simulink model "System_20220515"  (R2020b)
settings: Solver=ode4  StartTime=0.0  StopTime=inf  FixedStep=Ts  RelTol=1e-3  EnableMultiTasking=on
PreLoadFcn:
  | simulation_vars
PostLoadFcn:
  | simulation_vars
InitFcn:
  | simulation_vars
StartFcn:
  | simulation_vars
values from neighbouring files (symbols this model uses):
  ang_variance = 0.001*60    (= 0.06)    [simulation_vars.m]
  bus_va_seed = abs(round(1000*randn(73,1)))    [simulation_vars.m]
  bus_vm_seed = abs(round(1000*randn(73,1)))    [simulation_vars.m]
  event_time_end = event_time_start + 5/60    (= 10000.0833333)    [simulation_vars.m]
  event_time_start = 10000    [simulation_vars.m]
  line_iang0_seed = abs(round(1000*randn(104,1)))    [simulation_vars.m]
  line_iang1_seed = abs(round(1000*randn(104,1)))    [simulation_vars.m]
  line_imag0_seed = abs(round(1000*randn(104,1)))    [simulation_vars.m]
  line_imag1_seed = abs(round(1000*randn(104,1)))    [simulation_vars.m]
  mag_variance = 0.0005    [simulation_vars.m]
  spoof_lower_limit = -pi()/9    [simulation_vars.m]
  spoof_upper_limit = pi()/9    [simulation_vars.m]
  Ts = 0.001    [simulation_vars.m]
  xf_iang0_seed = abs(round(1000*randn(16,1)))    [simulation_vars.m]
  xf_iang1_seed = abs(round(1000*randn(16,1)))    [simulation_vars.m]
  xf_imag0_seed = abs(round(1000*randn(16,1)))    [simulation_vars.m]
  xf_imag1_seed = abs(round(1000*randn(16,1)))    [simulation_vars.m]
undefined symbols (not defined in the file or in its folder): en_spoofing_attack
libraries: rtlab x210, simulink x21, opal_lib x1, rtlab_phasor x1, rtio_spectracom x1
(part 1 of 4)
Description:
  | Model of a simple control system for use iin training.
settings Model: Creator=Paul Baracos  LastModifiedBy=sudo
settings DataIOCC: LimitDataPoints=on  SaveFormat=Array  SignalLoggingSaveFormat=ModelDataLogs  SaveOutput=off  SaveTime=off  ReturnWorkspaceOutputs=off  SignalLoggingName=sigsOut
settings OptimizationCC: BlockReduction=off  BooleanDataType=off  OptimizeBlockIOStorage=off  BufferReuse=off  ExpressionFolding=off  LocalBlockOutputs=off  InitFltsAndDblsToZero=on  LifeSpan=inf
settings DebuggingCC: SaveWithParameterizedLinksMsg=none  UnderspecifiedInitializationDetection=Classic  MergeDetectMultiDrivingBlocksExec=none  SignalResolutionControl=TryResolveAllWithWarning  MultiTaskDSMMsg=warning  MultiTaskCondExecSysMsg=none  FcnCallInpInsideContextMsg=warning  SFUnexpectedBacktrackingDiag=warning  SFNoUnconditionalDefaultTransitionDiag=warning  SFExecutionAtInitializationDiag=none  ArithmeticOperatorsInVariantConditions=warning
settings HardwareCC: ProdBitPerPointer=32  ProdBitPerSizeT=32  ProdBitPerPtrDiffT=32  ProdLargestAtomicFloat=None  ProdIntDivRoundTo=Undefined  ProdEndianess=Unspecified  ProdWordSize=32  ProdHWDeviceType=32-bit Generic  TargetUnknown=on
settings ModelReferenceCC: PropagateSignalLabelsOutOfModel=off
settings SFSimCC: SimUseLocalCustomCode=off  CustomCodeUndefinedFunction=UseInterfaceOnly
settings RTWCC: RTWUseLocalCustomCode=off
settings CodeAppCC: StateflowObjectComments=on
settings GRTTargetCC: TargetFcnLib=ansi_tfl_tmw.mat  TargetLangStandard=C89/C90 (ANSI)  CombineOutputUpdateFcns=off  GRTInterface=on
settings ConfigComp: CovMetricSettings=dw  CovSaveCumulativeToWorkspaceVar=on  CovSaveSingleToWorkspaceVar=on  CovExternalEMLEnable=off

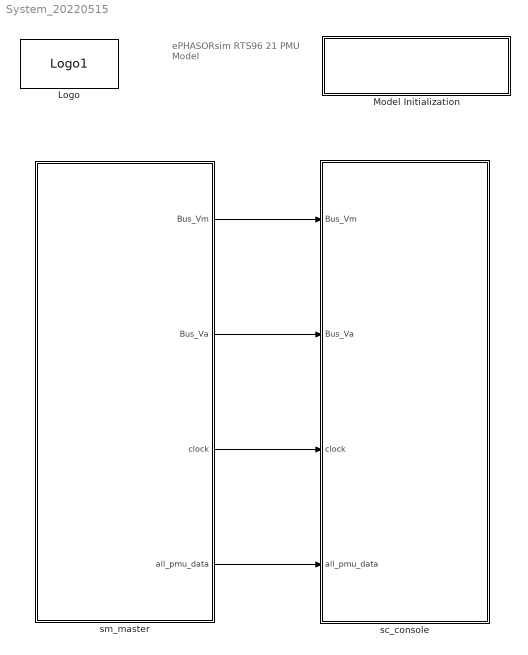
== system System_20220515 ==
  note: ePHASORsim
      | RTS96
      | 21 PMU Model
  Logo : opal_lib/Logo1  vide=[]
  Model Initialization : Subsystem  mask(Model Functions){InitFcnX=simulation_vars, prel=on, posl=on, inif=on, strf=on}
      mask prompts: InitFcnX "Initialisation"; prel "Preload Function"; posl "PostLoad Function"; inif "InitFcn"; strf "StartFcn"
      mask init:
      | currentBlock = gcb;
      | root = bdroot(currentBlock);
      | 
      | if ~strcmp(get_param(root,'BlockDiagramType'),'library')
      |     if prel==1
      |         set_param(root, 'PreLoadFcn', InitFcnX);
      |     else
      |         set_param(root, 'PreLoadFcn', '');
      |     end
      |     if inif==1
      |         set_param(root, 'InitFcn', InitFcnX);
      |     else
      |         set_param(root, 'InitFcn', '');
      |     end
      |     if strf==1
      |         set_param(root, 'StartFcn', InitFcnX);
      |     else
      |         set_param(root, 'StartFcn', '');
      |     end
      |     if posl==1
      |         set_param(root, 'PostLoadFcn', InitFcnX);
      |     else
      |         set_param(root, 'PostLoadFcn', '');
      |     end
      | end
      | 
      | pos = get_param(currentBlock, 'Position');
      | width = pos(3) - pos(1); height = pos(4) - pos(2);
      | txt = [ upper(root) '\n' '- InitFcn. . . . . '  get_param(root, 'InitFcn') ];
      settings: CopyFcn=set_param(gcb,'LinkStatus','none')
      mask Display: text(5, height*0.5, txt, 'horizontalAlignment', 'left', 'verticalAlignment', 'middle') ;
  sc_console : Subsystem
  sm_master : Subsystem
  wires:
  sm_master/1(Bus_Vm) -> sc_console/1(Bus_Vm)
  sm_master/3(clock) -> sc_console/3(clock)
  sm_master/4(all_pmu_data) -> sc_console/4(all_pmu_data)
  sm_master/2(Bus_Va) -> sc_console/2(Bus_Va)

== system System_20220515/Model Initialization ==

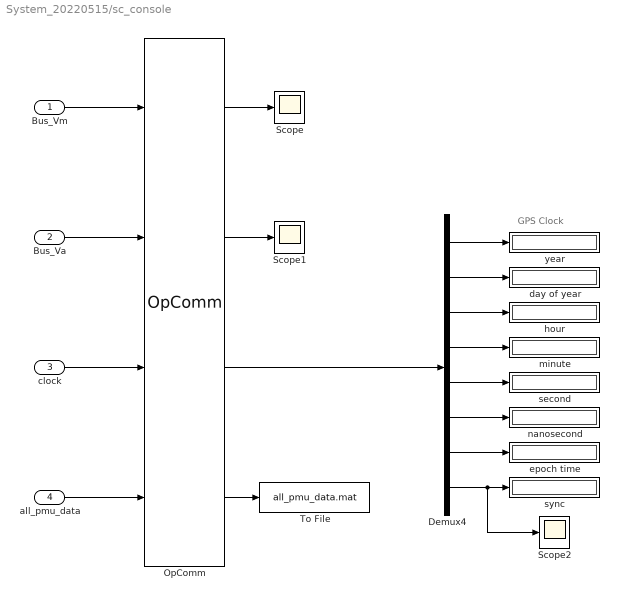
== system System_20220515/sc_console ==
  note: GPS Clock
  Bus_Vm : Inport
  Bus_Va : Inport  Port=2
  clock : Inport  Port=3
  all_pmu_data : Inport  Port=4
  Demux4 : Demux  Outputs=8
  OpComm : rtlab/OpComm  nbport=4  groupe_acq=1  subsys_rate=0  st=0  Synchronization=on  Interpolation=on  Threshold=1.0  Missed_Data=off  Sim_Time=off  Samples=off  dynSigOut=off  from_console=0  warning_done=off  writeOpCommFile=off  Offset=off
      settings: SourceProductName=RT-LAB
  Scope : Scope
  Scope1 : Scope
  Scope2 : Scope
  To File : ToFile  Filename=all_pmu_data.mat  SaveFormat=Timeseries
  day of year : Display
  epoch time : Display
  hour : Display
  minute : Display
  nanosecond : Display
  second : Display
  sync : Display
  year : Display
  wires:
  Bus_Vm/1 -> OpComm/1
  OpComm/1 -> Scope/1
  Demux4/3 -> hour/1
  Demux4/8 -> Scope2/1, sync/1
  Demux4/4 -> minute/1
  Demux4/2 -> day of year/1
  Demux4/5 -> second/1
  Demux4/6 -> nanosecond/1
  Demux4/1 -> year/1
  Demux4/7 -> epoch time/1
  all_pmu_data/1 -> OpComm/4
  clock/1 -> OpComm/3
  Bus_Va/1 -> OpComm/2
  OpComm/4 -> To File/1
  OpComm/3 -> Demux4/1
  OpComm/2 -> Scope1/1

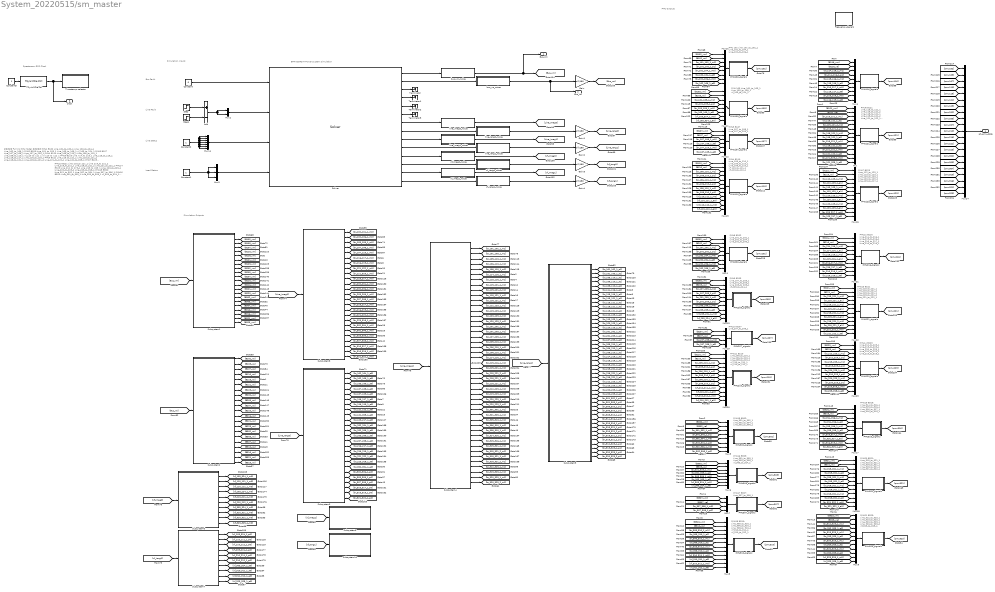
== system System_20220515/sm_master ==
  note: PMU13 B221
      | Line_215_to_221_1
      | Line_215_to_221_2
      | Line_218_to_221_1
      | Line_218_to_221_2
      | Line_221_to_222_1
      |
      | PMU14 B223
      | Line_212_to_223_1
      | Line_213_to_223_1
      | Line_220_to_223_1
      | Line_220_to_223_2
      | Line_223_to_318_1
      |
      | PMU15 B302:
      | Line_301_to_302_1
      | Line_302_to_304_1
      | Line_302_to_306_1
      |
      | PMU16 B303:
      | Line_301_to_303_1
      | Line_303_to_309_1
      | xf_303_to_324_1
      |
      | PMU17 B307:
      | Line_307_to_308_1
      |
      | PMU18 B310:
      | Line_305_to_310_1
      | Line_306_to_310_1
      | Line_308_to_310_1
      | xf_310_to_311_1
      | xf_310_to_312_1
      |
      | PMU19 B316:
      | Line_314_to_316_1
      | Line_315_to_316_1
      | Line_316_to_317_1
      | Line_316_to_319_1
      |
      | PMU20 B321:
      | Line_315_to_321_1
      | Line_315_to_321_2
      | Line_318_to_321_1
      | Line_318_to_321_2
      | Line_321_to_322_1
      |
      | PMU21 B323:
      | Line_312_to_323_1
      | Line_313_to_323_1
      | Line_320_to_323_1
      | Line_320_to_323_2
      | xf_323_to_325_1
  note: PMU14 B223
      | Line_212_to_223_1
      | Line_213_to_223_1
      | Line_220_to_223_1
      | Line_220_to_223_2
      | Line_223_to_318_1
  note: PMU12 B216
      | Line_214_to_216_1
      | Line_215_to_216_1
      | Line_216_to_217_1
      | Line_216_to_219_1
  note: PMU11 B210
      | Line_205_to_210_1
      | Line_206_to_210_1
      | Line_208_to_210_1
      | xf_210_to_211_1
      | xf_210_to_212_1
  note: PMU10 B207
      | Line_207_to_208_1
  note: PMU9 B203
      | Line_107_to_203_1
      | Line_201_to_203_1
      | Line_203_to_209_1
      | xf_203_to_224_1
  note: PMU8 B202
      | Line_201_to_202_1
      | LIne_202_to_204_1
      | Line_202_to_206_1
  note: PMU21 B323:
      | Line_312_to_323_1
      | Line_313_to_323_1
      | Line_320_to_323_1
      | Line_320_to_323_2
      | xf_323_to_325_1
  note: PMU20 B321:
      | Line_315_to_321_1
      | Line_315_to_321_2
      | Line_318_to_321_1
      | Line_318_to_321_2
      | Line_321_to_322_1
  note: PMU19 B316:
      | Line_314_to_316_1
      | Line_315_to_316_1
      | Line_316_to_317_1
      | Line_316_to_319_1
  note: PMU18 B310:
      | Line_305_to_310_1
      | Line_306_to_310_1
      | Line_308_to_310_1
      | xf_310_to_311_1
      | xf_310_to_312_1
  note: PMU17 B307:
      | Line_307_to_308_1
  note: PMU16 B303:
      | Line_301_to_303_1
      | Line_303_to_309_1
      | xf_303_to_324_1
  note: PMU15 B302:
      | Line_301_to_302_1
      | Line_302_to_304_1
      | Line_302_to_306_1
  note: PMU 102
      | Line_101_to_102_1
      | Line_102_to_104_1
      | Line_102_to_106_1
  note: EPHASORSIM Power System Simulation
  note: Simulation Inputs
  note: Simulation Outputs
  note: PMU Outputs
  note: Spectracom GPS Clock
  note: ##### Full 21 PMU Model #####
      | PMU1 B102
      | Line_101_to_102_1
      | Line_102_to_104_1
      | Line_102_to_106_1
      |
      | PMU2 B103
      | Line_101_to_103_1
      | Line_103_to_109_1
      | xf_103_to_124_1
      |
      | PMU3 B107
      | Line_107_to_108_1
      | Line_107_to_203_1
      |
      | PMU4 B110
      | Line_105_to_110_1
      | Line_106_to_110_1
      | Line_108_to_110_1
      | xf_110_to_111_1
      | xf_110_to_112_1
      |
      | PMU5 B116
      | Line_114_to_116_1
      | Line_115_to_116_1
      | Line_116_to_117_1
      | Line_116_to_119_1
      |
      | PMU6 B121
      | Line_115_to_121_1
      | Line_115_to_121_2
      | Line_118_to_121_1
      | Line_118_to_121_2
      | Line_121_to_122_1
      | Line_121_to_325_1
      |
      | PMU7 B123
      | Line_112_to_123_1
      | Line_113_to_123_1
      | Line_120_to_123_1
      | Line_120_to_123_2
      | Line_123_to_217_1
      |
      | PMU8 B202
      | Line_201_to_202_1
      | LIne_202_to_204_1
      | Line_202_to_206_1
      |
      | PMU9 B203
      | Line_201_to_203_1
      | Line_203_to_209_1
      | Line_107_to_203_1
      | xf_203_to_224_1
      |
      | PMU10 B207
      | Line_207_to_208_1
      |
      | PMU11 B210
      | Line_205_to_210_1
      | Line_206_to_210_1
      | Line_208_to_210_1
      | xf_210_to_211_1
      | xf_210_to_212_1
      |
      | PMU12 B216
      | Line_214_to_216_1
      | Line_215_to_216_1
      | Line_216_to_217_1
      | Line_216_to_219_1
  note: Bus Fault
  note: Line Fault
  note: Line Status
  note: Load Status
  note: PMU 103
      | Line_101_to_103_1
      | Line_103_to_109_1
      | xf_103_to_124_1
  note: PMU3 B107
      | Line_107_to_108_1
      | Line_107_to_203_1
  note: PMU4 B110
      | Line_105_to_110_1
      | Line_106_to_110_1
      | Line_108_to_110_1
      | xf_110_to_111_1
      | xf_110_to_112_1
  note: PMU6 B121
      | Line_115_to_121_1
      | Line_115_to_121_2
      | Line_118_to_121_1
      | Line_118_to_121_2
      | Line_121_to_122_1
      | Line_121_to_325_1
  note: PMU7 B123
      | Line_112_to_123_1
      | Line_113_to_123_1
      | Line_120_to_123_1
      | Line_120_to_123_2
      | Line_123_to_217_1
  note: PMU13 B221
      | Line_215_to_221_1
      | Line_215_to_221_2
      | Line_218_to_221_1
      | Line_218_to_221_2
      | Line_221_to_222_1
  Add : Sum  Inputs=+-
  Constant : Constant  Value=0
  Constant1 : Constant
  Constant2 : Constant
  Constant3 : Constant
  Frequency_signals : Subsystem
  Gain{,1..4} (5 alike) : Gain  Gain=pi()/180
  Mux : Mux  Inputs=14
  Mux{1,5..6,10..11} (5 alike) : Mux  Inputs=8
  Mux12 : Mux  Inputs=6
  Mux{4,13,17,21} (4 alike) : Mux  Inputs=10
  Mux14 : Mux  Inputs=7
  Mux{8..9,15..16,18,20,22..23} (8 alike) : Mux  Inputs=12
  Mux19 : Mux
  Mux2 : Mux  Inputs=2
  Mux24 : Mux  Inputs=21
  Mux3 : Mux  Inputs=3
  Mux7 : Mux
  PMU102_signals : Subsystem
  PMU103_signals : Subsystem
  PMU107_signals : Subsystem
  PMU110_signals : Subsystem
  PMU116_signals : Subsystem
  PMU121_signals : Subsystem
  PMU123_signals : Subsystem
  PMU202_signals : Subsystem
  PMU203_signals : Subsystem
  PMU207_signals : Subsystem
  PMU210_signals : Subsystem
  PMU216_signals : Subsystem
  PMU221_signals : Subsystem
  PMU223_signals : Subsystem
  PMU302_signals : Subsystem
  PMU303_signals : Subsystem
  PMU307_signals : Subsystem
  PMU310_signals : Subsystem
  PMU316_signals : Subsystem
  PMU321_signals : Subsystem
  PMU323_signals : Subsystem
  Solver : rtlab_phasor/Solver  epname=System  extension=PSS/e Ver. 32  use_udb=off  xls='RTS96_pins_simple_v2.xls'  raw='RTS96_psse_stable.raw'  dyr='Dynamics.dyr'  fmu2builtin=off  cyme='typical.sxst'  cyme_pf=''  cyme_unbalanced=on  powerfactory='network.dgs'  builtin=on  lazy_netlist=on  capidir='CAPI'  fmudir='FMU'  capiprefix=capicomp_  fmuprefix=fmucomp_  logging=off  sim_mode=Power-flow and dynamic simulation  dt=Ts  pf_init_method=From input data  pf_tol_v=0.00000001  pf_max_it=100  pf_smart_start=off  pf_flat_start=off  pf_export=off  pfrequest=off  pf_then_dyn=on  np=1  exporty=off  optim_threads=on  perflog_on=off  script_activate_postinit=off  script_postinit_name=''
  Step : Step  Time=event_time_start  SampleTime=0
  Step1 : Step  Time=event_time_end  SampleTime=0
  Subsystem1 : Subsystem
  Subsystem10 : Subsystem
  Subsystem2 : Subsystem
  Subsystem3 : Subsystem
  Subsystem4 : Subsystem
  Subsystem5 : Subsystem
  Subsystem6 : Subsystem
  Subsystem7 : Subsystem
  Subsystem8 : Subsystem
  Subsystem9 : Subsystem
  TSync PCIe Ctrl : rtio_spectracom/TSync PCIe Ctrl  devIx=0  holdover_timeout=5  timestamp_en=on  set_time_en=off  ts_wo_sync_opt=UTC 0
  Terminator{,1..3} (4 alike) : Terminator
  Timestamp selector : Subsystem
  bus_va_noise : Subsystem
  bus_vm_noise : Subsystem
  line_iang0_noise : Subsystem
  line_iang1_noise : Subsystem
  line_imag0_noise : Subsystem
  line_imag1_noise : Subsystem
  xf_iang0_noise : Subsystem
  xf_iang1_noise : Subsystem
  xf_imag0_noise : Subsystem
  xf_imag1_noise : Subsystem
  Bus_Vm : Outport  VectorParamsAs1DForOutWhenUnconnected=off
  Bus_Va : Outport  Port=2
  clock : Outport  Port=3
  all_pmu_data : Outport  Port=4
  wires:
  Solver/2 -> bus_va_noise/1(In1)
  Solver/10 -> line_iang1_noise/1(In1)
  Solver/8 -> line_iang0_noise/1(In1)
  Solver/12 -> xf_iang0_noise/1(In1)
  Subsystem1/5(B116_Vmag) -> [B116_vm]
  Subsystem1/16(B303_Vmag) -> [B303_vm]
  Subsystem1/6(B121_Vmag) -> [B121_vm]
  Subsystem1/17(B307_Vmag) -> [B307_vm]
  Subsystem1/15(B302_Vmag) -> [B302_vm]
  Subsystem1/18(B310_Vmag) -> [B310_vm]
  Subsystem1/21(B323_Vmag) -> [B323_vm]
  Subsystem2/15(B302_Vang) -> [B302_va]
  Subsystem2/6(B121_Vang) -> [B121_va]
  Subsystem2/5(B116_Vang) -> [B116_va]
  Subsystem2/16(B303_Vang) -> [B303_va]
  Subsystem2/17(B307_Vang) -> [B307_va]
  Subsystem2/18(B310_Vang) -> [B310_va]
  Subsystem2/21(B323_Vang) -> [B323_va]
  Subsystem4/6(Line_114_to_116_1_mag) -> [br_114_116_1_m1]
  Subsystem4/7(Line_115_to_116_1_mag) -> [br_115_116_1_m1]
  Subsystem8/6(Line_116_to_117_1_mag) -> [br_116_117_1_m0]
  Subsystem8/7(Line_116_to_119_1_mag) -> [br_116_119_1_m0]
  Subsystem4/8(Line_115_to_121_1_mag) -> [br_115_121_1_m1]
  Subsystem4/9(Line_115_to_121_2_mag) -> [br_115_121_2_m1]
  Subsystem4/10(Line_118_to_121_1_mag) -> [br_118_121_1_m1]
  Subsystem4/11(Line_118_to_121_2_mag) -> [br_118_121_2_m1]
  Subsystem8/8(Line_121_to_122_1_mag) -> [br_121_122_1_m0]
  Subsystem8/9(Line_121_to_325_1_mag) -> [br_121_325_1_m0]
  Subsystem4/32(Line_301_to_302_1_mag) -> [br_301_302_1_m1]
  Subsystem8/19(Line_302_to_304_1_mag) -> [br_302_304_1_m0]
  Subsystem8/20(Line_302_to_306_1_mag) -> [br_302_306_1_m0]
  Subsystem4/33(Line_301_to_303_1_mag) -> [br_301_303_1_m1]
  Subsystem8/21(Line_303_to_309_1_mag) -> [br_303_309_1_m0]
  Subsystem8/22(Line_307_to_308_1_mag) -> [br_307_308_1_m0]
  Subsystem4/34(Line_305_to_310_1_mag) -> [br_305_310_1_m1]
  Subsystem4/35(Line_306_to_310_1_mag) -> [br_306_310_1_m1]
  Subsystem4/36(Line_308_to_310_1_mag) -> [br_308_310_1_m1]
  Subsystem4/43(Line_312_to_323_1_mag) -> [br_312_323_1_m1]
  Subsystem4/44(Line_313_to_323_1_mag) -> [br_313_323_1_m1]
  Subsystem4/45(Line_320_to_323_1_mag) -> [br_320_323_1_m1]
  Subsystem4/46(Line_320_to_323_2_mag) -> [br_320_323_2_m1]
  Subsystem6/7(xf_303_to_324_1_mag) -> [xf_303_324_1_m0]
  Subsystem6/8(xf_310_to_311_1_mag) -> [xf_310_311_1_m0]
  Subsystem6/9(xf_310_to_312_1_mag) -> [xf_310_312_1_m0]
  Subsystem6/10(xf_323_to_325_1_mag) -> [xf_323_325_1_m0]
  Solver/14 -> xf_iang1_noise/1(In1)
  Constant/1 -> Solver/1
  Step/1 -> Add/1
  Step1/1 -> Add/2
  Mux2/1 -> Solver/2
  Add/1 -> Mux2/1, Mux2/2
  Mux3/1 -> Solver/4
  Constant1/1 -> Mux3/3, Mux3/1, Mux3/2
  Mux14/1 -> Solver/3
  [B116_vm] -> Mux4/1
  [B116_va] -> Mux4/2
  [br_114_116_1_m1] -> Mux4/3
  [br_114_116_1_a1] -> Mux4/4
  [br_115_116_1_m1] -> Mux4/5
  [br_115_116_1_a1] -> Mux4/6
  [br_116_117_1_m0] -> Mux4/7
  [br_116_117_1_a0] -> Mux4/8
  [br_116_119_1_m0] -> Mux4/9
  [br_116_119_1_a0] -> Mux4/10
  [B121_vm] -> Mux/1
  [B121_va] -> Mux/2
  [br_115_121_1_m1] -> Mux/3
  Mux/1 -> PMU121_signals/1(In1)
  [br_115_121_1_a1] -> Mux/4
  [br_115_121_2_m1] -> Mux/5
  [br_115_121_2_a1] -> Mux/6
  [br_118_121_1_m1] -> Mux/7
  [br_118_121_1_a1] -> Mux/8
  [br_118_121_2_m1] -> Mux/9
  [br_118_121_2_a1] -> Mux/10
  [br_121_122_1_m0] -> Mux/11
  [br_121_122_1_a0] -> Mux/12
  [br_121_325_1_m0] -> Mux/13
  [br_121_325_1_a0] -> Mux/14
  Mux5/1 -> PMU302_signals/1(In1)
  [B302_vm] -> Mux5/1
  [B302_va] -> Mux5/2
  [br_301_302_1_m1] -> Mux5/3
  [br_301_302_1_a1] -> Mux5/4
  [br_302_304_1_m0] -> Mux5/5
  [br_302_304_1_a0] -> Mux5/6
  [br_302_306_1_m0] -> Mux5/7
  [br_302_306_1_a0] -> Mux5/8
  [B303_vm] -> Mux6/1
  [B303_va] -> Mux6/2
  [br_301_303_1_m1] -> Mux6/3
  [br_301_303_1_a1] -> Mux6/4
  [br_303_309_1_m0] -> Mux6/5
  [br_303_309_1_a0] -> Mux6/6
  [xf_303_324_1_m0] -> Mux6/7
  [xf_303_324_1_a0] -> Mux6/8
  Mux6/1 -> PMU303_signals/1(In1)
  [B307_vm] -> Mux7/1
  [B307_va] -> Mux7/2
  [br_307_308_1_m0] -> Mux7/3
  [br_307_308_1_a0] -> Mux7/4
  Mux7/1 -> PMU307_signals/1(In1)
  [B310_vm] -> Mux8/1
  [B310_va] -> Mux8/2
  [br_305_310_1_m1] -> Mux8/3
  [br_305_310_1_a1] -> Mux8/4
  [br_306_310_1_m1] -> Mux8/5
  [br_306_310_1_a1] -> Mux8/6
  [br_308_310_1_m1] -> Mux8/7
  [br_308_310_1_a1] -> Mux8/8
  [xf_310_311_1_m0] -> Mux8/9
  [xf_310_311_1_a0] -> Mux8/10
  [xf_310_312_1_m0] -> Mux8/11
  [xf_311_312_1_a0] -> Mux8/12
  Mux8/1 -> PMU310_signals/1(In1)
  [B323_vm] -> Mux9/1
  [B323_va] -> Mux9/2
  [br_312_323_1_m1] -> Mux9/3
  [br_312_323_1_a1] -> Mux9/4
  [br_313_323_1_m1] -> Mux9/5
  [br_313_323_1_a1] -> Mux9/6
  [br_320_323_1_m1] -> Mux9/7
  [br_320_323_1_a1] -> Mux9/8
  [br_320_323_2_m1] -> Mux9/9
  [br_320_323_2_a1] -> Mux9/10
  [xf_323_325_1_m0] -> Mux9/11
  [xf_323_325_1_a0] -> Mux9/12
  Mux9/1 -> PMU323_signals/1(In1)
  PMU121_signals/1(Out1) -> [pmu121]
  PMU302_signals/1(Out1) -> [pmu302]
  PMU303_signals/1(Out1) -> [pmu303]
  PMU307_signals/1(Out1) -> [pmu307]
  PMU310_signals/1(Out1) -> [pmu310]
  PMU323_signals/1(Out1) -> [pmu323]
  PMU116_signals/1(Out1) -> [pmu116]
  Mux4/1 -> PMU116_signals/1(In1)
  TSync PCIe Ctrl/1 -> clock/1, Timestamp selector/1(ts_in)
  Constant3/1 -> TSync PCIe Ctrl/1
  Constant2/1 -> Mux14/5, Mux14/7, Mux14/6, Mux14/1, Mux14/2, Mux14/3, Mux14/4
  Solver/3 -> Terminator/1
  Solver/4 -> Terminator1/1
  Solver/5 -> Terminator2/1
  Solver/6 -> Terminator3/1
  Subsystem1/1(B102_Vmag) -> [B102_vm]
  [B102_vm] -> Mux10/1
  Subsystem2/1(B102_Vang) -> [B102_va]
  [B102_va] -> Mux10/2
  Mux10/1 -> PMU102_signals/1(In1)
  PMU102_signals/1(Out1) -> [pmu102]
  Subsystem4/1(Line_101_to_102_1_mag) -> [br_101_102_1_m1]
  [br_101_102_1_m1] -> Mux10/3
  [br_101_102_1_a1] -> Mux10/4
  Subsystem8/2(Line_102_to_106_1_mag) -> [br_102_106_1_m0]
  Subsystem8/1(Line_102_to_104_1_mag) -> [br_102_104_1_m0]
  [br_102_104_1_m0] -> Mux10/5
  [br_102_106_1_m0] -> Mux10/7
  Gain1/1 -> [Line_Iang0]
  [Line_Imag0] -> Subsystem8/1(Imag0)
  [Line_Iang0] -> Subsystem3/1(Iang0)
  Gain2/1 -> [Line_Iang1]
  [Line_Imag1] -> Subsystem4/1(Imag1)
  [Line_Iang1] -> Subsystem5/1(Iang1)
  [xf_Imag0] -> Subsystem6/1(Imag0)
  Gain3/1 -> [xf_Iang0]
  [xf_Iang0] -> Subsystem7/1(Iang0)
  [xf_Imag1] -> Subsystem9/1(Imag1)
  Gain4/1 -> [xf_Iang1]
  [Bus_vm] -> Subsystem1/1(bus_vm)
  Gain/1 -> [Bus_va]
  [Bus_va] -> Subsystem2/1(bus_va)
  Subsystem3/6(Line_116_to_117_1_ang) -> [br_116_117_1_a0]
  Subsystem3/7(Line_116_to_119_1_ang) -> [br_116_119_1_a0]
  Subsystem3/8(Line_121_to_122_1_ang) -> [br_121_122_1_a0]
  Subsystem3/9(Line_121_to_325_1_ang) -> [br_121_325_1_a0]
  Subsystem3/22(Line_307_to_308_1_ang) -> [br_307_308_1_a0]
  Subsystem3/21(Line_303_to_309_1_ang) -> [br_303_309_1_a0]
  Subsystem3/20(Line_302_to_306_1_ang) -> [br_302_306_1_a0]
  Subsystem3/19(Line_302_to_304_1_ang) -> [br_302_304_1_a0]
  Subsystem3/2(Line_102_to_106_1_ang) -> [br_102_106_1_a0]
  Subsystem3/1(Line_102_to_104_1_ang) -> [br_102_104_1_a0]
  [br_102_104_1_a0] -> Mux10/6
  [br_102_106_1_a0] -> Mux10/8
  Subsystem1/2(B103_Vmag) -> [B103_vm]
  Subsystem2/2(B103_Vang) -> [B103_va]
  Subsystem8/3(Line_103_to_109_1_mag) -> [br_103_109_1_m0]
  Subsystem3/3(Line_103_to_109_1_ang) -> [br_103_109_1_a0]
  [xf_Iang1] -> Subsystem10/1(Iang1)
  Subsystem7/7(xf_303_to_324_1_ang) -> [xf_303_324_1_a0]
  Subsystem7/8(xf_310_to_311_1_ang) -> [xf_310_311_1_a0]
  Subsystem7/9(xf_310_to_312_1_ang) -> [xf_311_312_1_a0]
  Subsystem7/10(xf_323_to_325_1_ang) -> [xf_323_325_1_a0]
  Subsystem4/2(Line_101_to_103_1_mag) -> [br_101_103_1_m1]
  Subsystem5/1(Line_101_to_102_1_ang) -> [br_101_102_1_a1]
  Subsystem5/6(Line_114_to_116_1_ang) -> [br_114_116_1_a1]
  Subsystem5/7(Line_115_to_116_1_ang) -> [br_115_116_1_a1]
  Subsystem5/9(Line_115_to_121_2_ang) -> [br_115_121_2_a1]
  Subsystem5/8(Line_115_to_121_1_ang) -> [br_115_121_1_a1]
  Subsystem5/10(Line_118_to_121_1_ang) -> [br_118_121_1_a1]
  Subsystem5/11(Line_118_to_121_2_ang) -> [br_118_121_2_a1]
  Subsystem5/32(Line_301_to_302_1_ang) -> [br_301_302_1_a1]
  Subsystem5/33(Line_301_to_303_1_ang) -> [br_301_303_1_a1]
  Subsystem5/34(Line_305_to_310_1_ang) -> [br_305_310_1_a1]
  Subsystem5/35(Line_306_to_310_1_ang) -> [br_306_310_1_a1]
  Subsystem5/36(Line_308_to_310_1_ang) -> [br_308_310_1_a1]
  Subsystem5/46(Line_320_to_323_2_ang) -> [br_320_323_2_a1]
  Subsystem5/45(Line_320_to_323_1_ang) -> [br_320_323_1_a1]
  Subsystem5/44(Line_313_to_323_1_ang) -> [br_313_323_1_a1]
  Subsystem5/43(Line_312_to_323_1_ang) -> [br_312_323_1_a1]
  Subsystem5/2(Line_101_to_103_1_ang) -> [br_101_103_1_a1]
  [br_101_103_1_m1] -> Mux11/3
  [br_101_103_1_a1] -> Mux11/4
  [br_103_109_1_m0] -> Mux11/5
  [br_103_109_1_a0] -> Mux11/6
  [B103_va] -> Mux11/2
  [B103_vm] -> Mux11/1
  Mux11/1 -> PMU103_signals/1(In1)
  PMU103_signals/1(Out1) -> [pmu103]
  Subsystem1/3(B107_Vmag) -> [B107_vm]
  Subsystem2/3(B107_Vang) -> [B107_va]
  Subsystem8/4(Line_107_to_108_1_mag) -> [br_107_108_1_m0]
  Subsystem3/4(Line_107_to_108_1_ang) -> [br_107_108_1_a0]
  Subsystem8/5(Line_107_to_203_1_mag) -> [br_107_123_1_m0]
  Subsystem3/5(Line_107_to_203_1_ang) -> [br_107_123_1_a0]
  [br_107_123_1_a0] -> Mux12/6
  [br_107_123_1_m0] -> Mux12/5
  [br_107_108_1_a0] -> Mux12/4
  [br_107_108_1_m0] -> Mux12/3
  [B107_va] -> Mux12/2
  [B107_vm] -> Mux12/1
  Mux12/1 -> PMU107_signals/1(In1)
  PMU107_signals/1(Out1) -> [pmu107]
  Subsystem6/1(xf_103_to_124_1_mag) -> [xf_103_324_1_m0]
  [xf_103_324_1_m0] -> Mux11/7
  Subsystem7/1(xf_103_to_124_1_ang) -> [xf_103_324_1_a0]
  [xf_103_324_1_a0] -> Mux11/8
  Subsystem1/4(B110_Vmag) -> [B110_vm]
  Subsystem2/4(B110_Vang) -> [B110_va]
  Subsystem4/3(Line_105_to_110_1_mag) -> [br_105_110_1_m1]
  Subsystem4/4(Line_106_to_110_1_mag) -> [br_106_110_1_m1]
  Subsystem4/5(Line_108_to_110_1_mag) -> [br_108_110_1_m1]
  Subsystem6/2(xf_110_to_111_1_mag) -> [xf_110_111_1_m0]
  Subsystem6/3(xf_110_to_112_1_mag) -> [xf_110_112_1_m0]
  Subsystem7/2(xf_110_to_111_1_ang) -> [xf_110_111_1_a0]
  Subsystem7/3(xf_110_to_112_1_ang) -> [xf_110_112_1_a0]
  Subsystem5/3(Line_105_to_110_1_ang) -> [br_105_110_1_a1]
  Subsystem5/4(Line_106_to_110_1_ang) -> [br_106_110_1_a1]
  Subsystem5/5(Line_108_to_110_1_ang) -> [br_108_110_1_a1]
  [br_108_110_1_m1] -> Mux15/7
  [xf_110_112_1_a0] -> Mux15/12
  Mux15/1 -> PMU110_signals/1(Input)
  [B110_va] -> Mux15/2
  [br_106_110_1_a1] -> Mux15/6
  PMU110_signals/1(Output) -> [pmu110]
  [br_105_110_1_m1] -> Mux15/3
  [xf_110_111_1_m0] -> Mux15/9
  [B110_vm] -> Mux15/1
  [br_108_110_1_a1] -> Mux15/8
  [xf_110_112_1_m0] -> Mux15/11
  [br_105_110_1_a1] -> Mux15/4
  [xf_110_111_1_a0] -> Mux15/10
  [br_106_110_1_m1] -> Mux15/5
  Subsystem1/7(B123_Vmag) -> [B123_vm]
  Subsystem2/7(B123_Vang) -> [B123_va]
  [B123_va] -> Mux16/2
  [B123_vm] -> Mux16/1
  PMU123_signals/1(Out1) -> [pmu123]
  Mux16/1 -> PMU123_signals/1(In1)
  Subsystem8/10(Line_123_to_217_1_mag) -> [br_123_217_1_m0]
  [br_123_217_1_m0] -> Mux16/11
  Subsystem3/10(Line_123_to_217_1_ang) -> [br_123_217_1_a0]
  [br_123_217_1_a0] -> Mux16/12
  Subsystem4/12(Line_112_to_123_1_mag) -> [br_112_123_1_m1]
  Subsystem4/13(Line_113_to_123_1_mag) -> [br_113_123_1_m1]
  Subsystem4/14(Line_120_to_123_1_mag) -> [br_120_123_1_m1]
  Subsystem4/15(Line_120_to_123_2_mag) -> [br_120_123_2_m1]
  [br_113_123_1_m1] -> Mux16/5
  [br_112_123_1_m1] -> Mux16/3
  [br_120_123_1_m1] -> Mux16/7
  [br_120_123_2_m1] -> Mux16/9
  Subsystem5/12(Line_112_to_123_1_ang) -> [br_112_123_1_a1]
  Subsystem5/13(Line_113_to_123_1_ang) -> [br_113_123_1_a1]
  Subsystem5/14(Line_120_to_123_1_ang) -> [br_120_123_1_a1]
  Subsystem5/15(Line_120_to_123_2_ang) -> [br_120_123_2_a1]
  [br_120_123_2_a1] -> Mux16/10
  [br_120_123_1_a1] -> Mux16/8
  [br_113_123_1_a1] -> Mux16/6
  [br_112_123_1_a1] -> Mux16/4
  Subsystem1/19(B316_Vmag) -> [B316_vm]
  Subsystem1/20(B321_Vmag) -> [B321_vm]
  Subsystem1/8(B202_Vmag) -> [B202_vm]
  Subsystem1/9(B203_Vmag) -> [B203_vm]
  Subsystem1/10(B207_Vmag) -> [B207_vm]
  Subsystem1/11(B210_Vmag) -> [B210_vm]
  Subsystem1/12(B216_Vmag) -> [B216_vm]
  Subsystem1/13(B221_Vmag) -> [B221_vm]
  Subsystem1/14(B223_Vmag) -> [B223_vm]
  Subsystem2/8(B202_Vang) -> [B202_va]
  Subsystem2/9(B203_Vang) -> [B203_va]
  Subsystem2/10(B207_Vang) -> [B207_va]
  Subsystem2/11(B210_Vang) -> [B210_va]
  Subsystem2/12(B216_Vang) -> [B216_va]
  Subsystem2/13(B221_Vang) -> [B221_va]
  Subsystem2/14(B223_Vang) -> [B223_va]
  Subsystem2/19(B316_Vang) -> [B316_va]
  Subsystem2/20(B321_Vang) -> [B321_va]
  [B316_vm] -> Mux17/1
  [B316_va] -> Mux17/2
  Subsystem4/37(Line_314_to_316_1_mag) -> [br_314_316_1_m1]
  [br_314_316_1_m1] -> Mux17/3
  Subsystem4/38(Line_315_to_316_1_mag) -> [br_315_316_1_m1]
  [br_315_316_1_m1] -> Mux17/5
  Subsystem5/37(Line_314_to_316_1_ang) -> [br_314_316_1_a1]
  Subsystem5/38(Line_315_to_316_1_ang) -> [br_315_316_1_a1]
  [br_314_316_1_a1] -> Mux17/4
  [br_315_316_1_a1] -> Mux17/6
  Subsystem8/23(Line_316_to_317_1_mag) -> [br_316_317_1_m0]
  Subsystem8/24(Line_316_to_319_1_mag) -> [br_316_319_1_m0]
  Subsystem8/25(Line_321_to_322_1_mag) -> [br_321_322_1_m0]
  [br_316_319_1_m0] -> Mux17/9
  [br_316_317_1_m0] -> Mux17/7
  Subsystem3/25(Line_321_to_322_1_ang) -> [br_321_322_1_a0]
  Subsystem3/24(Line_316_to_319_1_ang) -> [br_316_319_1_a0]
  Subsystem3/23(Line_316_to_317_1_ang) -> [br_316_317_1_a0]
  [br_316_317_1_a0] -> Mux17/8
  [br_316_319_1_a0] -> Mux17/10
  PMU316_signals/1(Out1) -> [pmu316]
  Mux17/1 -> PMU316_signals/1(In1)
  Subsystem4/39(Line_315_to_321_1_mag) -> [br_315_321_1_m1]
  Subsystem4/40(Line_315_to_321_2_mag) -> [br_315_321_2_m1]
  Subsystem4/41(Line_318_to_321_1_mag) -> [br_318_321_1_m1]
  Subsystem4/42(Line_318_to_321_2_mag) -> [br_318_321_2_m1]
  [B321_vm] -> Mux18/1
  [B321_va] -> Mux18/2
  [br_315_321_1_m1] -> Mux18/3
  [br_315_321_2_m1] -> Mux18/5
  [br_318_321_1_m1] -> Mux18/7
  [br_318_321_2_m1] -> Mux18/9
  [br_321_322_1_m0] -> Mux18/11
  [br_321_322_1_a0] -> Mux18/12
  PMU321_signals/1(Out1) -> [pmu321]
  Mux18/1 -> PMU321_signals/1(In1)
  Subsystem5/39(Line_315_to_321_1_ang) -> [br_315_321_1_a1]
  Subsystem5/40(Line_315_to_321_2_ang) -> [br_315_321_2_a1]
  Subsystem5/41(Line_318_to_321_1_ang) -> [br_318_321_1_a1]
  Subsystem5/42(Line_318_to_321_2_ang) -> [br_318_321_2_a1]
  [br_318_321_2_a1] -> Mux18/10
  [br_318_321_1_a1] -> Mux18/8
  [br_315_321_2_a1] -> Mux18/6
  [br_315_321_1_a1] -> Mux18/4
  Subsystem6/4(xf_203_to_224_1_mag) -> [xf_203_224_1_m0]
  Subsystem6/5(xf_210_to_211_1_mag) -> [xf_210_211_1_m0]
  Subsystem6/6(xf_210_to_212_1_mag) -> [xf_210_212_1_m0]
  Subsystem7/4(xf_203_to_224_1_ang) -> [xf_203_224_1_a0]
  Subsystem7/5(xf_210_to_211_1_ang) -> [xf_210_211_1_a0]
  Subsystem7/6(xf_210_to_212_1_ang) -> [xf_210_212_1_a0]
  [B202_vm] -> Mux1/1
  [B202_va] -> Mux1/2
  Subsystem8/11(Line_202_to_204_1_mag) -> [br_202_204_1_m0]
  Subsystem8/12(Line_202_to_206_1_mag) -> [br_202_206_1_m0]
  Subsystem8/13(Line_203_to_209_1_mag) -> [br_203_209_1_m0]
  Subsystem8/14(Line_207_to_208_1_mag) -> [br_207_208_1_m0]
  Subsystem8/15(Line_216_to_217_1_mag) -> [br_216_217_1_m0]
  Subsystem8/16(Line_216_to_219_1_mag) -> [br_216_219_1_m0]
  Subsystem8/17(Line_221_to_222_1_mag) -> [br_221_222_1_m0]
  Subsystem8/18(Line_223_to_318_1_mag) -> [br_223_318_1_m0]
  Subsystem3/11(Line_202_to_204_1_ang) -> [br_202_204_1_a0]
  Subsystem3/12(Line_202_to_206_1_ang) -> [br_202_206_1_a0]
  Subsystem3/13(Line_203_to_209_1_ang) -> [br_203_209_1_a0]
  Subsystem3/14(Line_207_to_208_1_ang) -> [br_207_208_1_a0]
  Subsystem3/15(Line_216_to_217_1_ang) -> [br_216_217_1_a0]
  Subsystem3/16(Line_216_to_219_1_ang) -> [br_216_219_1_a0]
  Subsystem3/17(Line_221_to_222_1_ang) -> [br_221_222_1_a0]
  Subsystem3/18(Line_223_to_318_1_ang) -> [br_223_318_1_a0]
  Subsystem4/16(Line_201_to_202_1_mag) -> [br_201_202_1_m1]
  Subsystem4/17(Line_201_to_203_1_mag) -> [br_201_203_1_m1]
  Subsystem4/18(Line_107_to_203_1_mag) -> [br_107_203_1_m1]
  Subsystem4/19(Line_205_to_210_1_mag) -> [br_205_210_1_m1]
  Subsystem4/20(Line_206_to_210_1_mag) -> [br_206_210_1_m1]
  Subsystem4/21(Line_208_to_210_1_mag) -> [br_208_210_1_m1]
  Subsystem4/22(Line_214_to_216_1_mag) -> [br_214_216_1_m1]
  Subsystem4/23(Line_215_to_216_1_mag) -> [br_215_216_1_m1]
  Subsystem4/24(Line_215_to_221_1_mag) -> [br_215_221_1_m1]
  Subsystem4/25(Line_215_to_221_2_mag) -> [br_215_221_2_m1]
  Subsystem4/26(Line_218_to_221_1_mag) -> [br_218_221_1_m1]
  Subsystem4/27(Line_218_to_221_2_mag) -> [br_218_221_2_m1]
  Subsystem4/28(Line_212_to_223_1_mag) -> [br_212_223_1_m1]
  Subsystem4/29(Line_213_to_223_1_mag) -> [br_213_223_1_m1]
  Subsystem4/30(Line_220_to_223_1_mag) -> [br_220_223_1_m1]
  Subsystem4/31(Line_220_to_223_2_mag) -> [br_220_223_2_m1]
  Subsystem5/31(Line_220_to_223_2_ang) -> [br_220_223_2_a1]
  Subsystem5/30(Line_220_to_223_1_ang) -> [br_220_223_1_a1]
  Subsystem5/29(Line_213_to_223_1_ang) -> [br_213_223_1_a1]
  Subsystem5/28(Line_212_to_223_1_ang) -> [br_212_223_1_a1]
  Subsystem5/27(Line_218_to_221_2_ang) -> [br_218_221_2_a1]
  Subsystem5/26(Line_218_to_221_1_ang) -> [br_218_221_1_a1]
  Subsystem5/25(Line_215_to_221_2_ang) -> [br_215_221_2_a1]
  Subsystem5/24(Line_215_to_221_1_ang) -> [br_215_221_1_a1]
  Subsystem5/23(Line_215_to_216_1_ang) -> [br_215_216_1_a1]
  Subsystem5/22(Line_214_to_216_1_ang) -> [br_214_216_1_a1]
  Subsystem5/21(Line_208_to_210_1_ang) -> [br_208_210_1_a1]
  Subsystem5/20(Line_206_to_210_1_ang) -> [br_206_210_1_a1]
  Subsystem5/16(Line_201_to_202_1_ang) -> [br_201_202_1_a1]
  Subsystem5/17(Line_201_to_203_1_ang) -> [br_201_203_1_a1]
  Subsystem5/18(Line_107_to_203_1_ang) -> [br_107_203_1_a1]
  Subsystem5/19(Line_205_to_210_1_ang) -> [br_205_210_1_a1]
  [br_201_202_1_m1] -> Mux1/3
  [br_201_202_1_a1] -> Mux1/4
  [br_202_206_1_m0] -> Mux1/7
  [br_202_204_1_m0] -> Mux1/5
  [br_202_204_1_a0] -> Mux1/6
  [br_202_206_1_a0] -> Mux1/8
  Mux1/1 -> PMU202_signals/1(In1)
  PMU202_signals/1(Out1) -> [pmu202]
  [B203_vm] -> Mux13/1
  [B203_va] -> Mux13/2
  [br_107_203_1_m1] -> Mux13/3
  [br_107_203_1_a1] -> Mux13/4
  [br_201_203_1_m1] -> Mux13/5
  [br_201_203_1_a1] -> Mux13/6
  [br_203_209_1_m0] -> Mux13/7
  [br_203_209_1_a0] -> Mux13/8
  [xf_203_224_1_m0] -> Mux13/9
  [xf_203_224_1_a0] -> Mux13/10
  PMU203_signals/1(Out1) -> [pmu203]
  Mux13/1 -> PMU203_signals/1(In1)
  [br_207_208_1_a0] -> Mux19/4
  [br_207_208_1_m0] -> Mux19/3
  [B207_va] -> Mux19/2
  [B207_vm] -> Mux19/1
  PMU207_signals/1(Out1) -> [pmu207]
  Mux19/1 -> PMU207_signals/1(In1)
  [xf_210_212_1_a0] -> Mux20/12
  [xf_210_212_1_m0] -> Mux20/11
  [xf_210_211_1_a0] -> Mux20/10
  [xf_210_211_1_m0] -> Mux20/9
  [br_208_210_1_a1] -> Mux20/8
  [br_208_210_1_m1] -> Mux20/7
  [br_206_210_1_a1] -> Mux20/6
  [br_206_210_1_m1] -> Mux20/5
  [br_205_210_1_a1] -> Mux20/4
  [br_205_210_1_m1] -> Mux20/3
  [B210_va] -> Mux20/2
  [B210_vm] -> Mux20/1
  PMU210_signals/1(Output) -> [pmu210]
  Mux20/1 -> PMU210_signals/1(Input)
  [br_214_216_1_m1] -> Mux21/3
  [br_214_216_1_a1] -> Mux21/4
  [br_215_216_1_a1] -> Mux21/6
  [br_215_216_1_m1] -> Mux21/5
  [B216_va] -> Mux21/2
  [B216_vm] -> Mux21/1
  [br_216_217_1_m0] -> Mux21/7
  [br_216_217_1_a0] -> Mux21/8
  [br_216_219_1_m0] -> Mux21/9
  [br_216_219_1_a0] -> Mux21/10
  Mux21/1 -> PMU216_signals/1(In1)
  PMU216_signals/1(Out1) -> [pmu216]
  [br_218_221_1_a1] -> Mux22/8
  [br_215_221_1_a1] -> Mux22/4
  PMU221_signals/1(Out1) -> [pmu221]
  [br_218_221_1_m1] -> Mux22/7
  [br_215_221_1_m1] -> Mux22/3
  [br_221_222_1_m0] -> Mux22/11
  Mux22/1 -> PMU221_signals/1(In1)
  [br_215_221_2_a1] -> Mux22/6
  [B221_vm] -> Mux22/1
  [br_221_222_1_a0] -> Mux22/12
  [br_218_221_2_m1] -> Mux22/9
  [br_215_221_2_m1] -> Mux22/5
  [br_218_221_2_a1] -> Mux22/10
  [B221_va] -> Mux22/2
  [br_220_223_2_a1] -> Mux23/10
  [br_220_223_2_m1] -> Mux23/9
  [br_220_223_1_a1] -> Mux23/8
  [br_220_223_1_m1] -> Mux23/7
  [br_213_223_1_a1] -> Mux23/6
  [br_213_223_1_m1] -> Mux23/5
  [br_212_223_1_a1] -> Mux23/4
  [br_212_223_1_m1] -> Mux23/3
  [br_223_318_1_m0] -> Mux23/11
  [br_223_318_1_a0] -> Mux23/12
  [B223_va] -> Mux23/2
  [B223_vm] -> Mux23/1
  PMU223_signals/1(Output) -> [pmu223]
  Mux23/1 -> PMU223_signals/1(Input)
  [pmu102] -> Mux24/1
  [pmu103] -> Mux24/2
  [pmu107] -> Mux24/3
  [pmu110] -> Mux24/4
  [pmu116] -> Mux24/5
  [pmu121] -> Mux24/6
  [pmu123] -> Mux24/7
  [pmu202] -> Mux24/8
  [pmu203] -> Mux24/9
  [pmu207] -> Mux24/10
  [pmu210] -> Mux24/11
  [pmu216] -> Mux24/12
  [pmu221] -> Mux24/13
  [pmu223] -> Mux24/14
  [pmu302] -> Mux24/15
  [pmu303] -> Mux24/16
  [pmu307] -> Mux24/17
  [pmu310] -> Mux24/18
  [pmu316] -> Mux24/19
  [pmu321] -> Mux24/20
  [pmu323] -> Mux24/21
  Mux24/1 -> all_pmu_data/1
  bus_vm_noise/1(Bus_Vm) -> Bus_Vm/1, [Bus_vm]
  line_imag0_noise/1(Out1) -> [Line_Imag0]
  Solver/7 -> line_imag0_noise/1(In1)
  line_imag1_noise/1(Out1) -> [Line_Imag1]
  Solver/9 -> line_imag1_noise/1(In1)
  xf_imag0_noise/1(Out1) -> [xf_Imag0]
  Solver/11 -> xf_imag0_noise/1(In1)
  Solver/13 -> xf_imag1_noise/1(In1)
  xf_imag1_noise/1(Out1) -> [xf_Imag1]
  bus_va_noise/1(y) -> Bus_Va/1, Gain/1
  line_iang0_noise/1(y) -> Gain1/1
  line_iang1_noise/1(y) -> Gain2/1
  xf_iang0_noise/1(y) -> Gain3/1
  xf_iang1_noise/1(y) -> Gain4/1
  Solver/1 -> bus_vm_noise/1(In1)

== system System_20220515/sm_master/Frequency_signals ==
  FREQ DEVIATION : Constant  Value=0
  FREQ ROC : Constant  Value=0
  FREQ_DEV : rtlab/OpOutput  identifier_use=FREQ_DEV  identifier_hide=FREQ_DEV  nb_parents_identifier=0
      settings: SourceProductName=RT-LAB
  ROCOF : rtlab/OpOutput  identifier_use=ROCOF  identifier_hide=ROCOF  nb_parents_identifier=0
      settings: SourceProductName=RT-LAB
  wires:
  FREQ ROC/1 -> ROCOF/1
  FREQ DEVIATION/1 -> FREQ_DEV/1

== system System_20220515/sm_master/PMU102_signals ==
  In1 : Inport
  Demux : Demux  Outputs=8
  PMU102_I1a : rtlab/OpOutput  identifier_use=PMU102_I1a  identifier_hide=PMU102_I1a  nb_parents_identifier=0
      settings: SourceProductName=RT-LAB
  PMU102_I1m : rtlab/OpOutput  identifier_use=PMU102_I1m  identifier_hide=PMU102_I1m  nb_parents_identifier=0
      settings: SourceProductName=RT-LAB
  PMU102_I2a : rtlab/OpOutput  identifier_use=PMU102_I2a  identifier_hide=PMU102_I2a  nb_parents_identifier=0
      settings: SourceProductName=RT-LAB
  PMU102_I2m : rtlab/OpOutput  identifier_use=PMU102_I2m  identifier_hide=PMU102_I2m  nb_parents_identifier=0
      settings: SourceProductName=RT-LAB
  PMU102_I3a : rtlab/OpOutput  identifier_use=PMU102_I3a  identifier_hide=PMU102_I3a  nb_parents_identifier=0
      settings: SourceProductName=RT-LAB
  PMU102_I3m : rtlab/OpOutput  identifier_use=PMU102_I3m  identifier_hide=PMU102_I3m  nb_parents_identifier=0
      settings: SourceProductName=RT-LAB
  PMU102_Va : rtlab/OpOutput  identifier_use=PMU102_Va  identifier_hide=PMU102_Va  nb_parents_identifier=0
      settings: SourceProductName=RT-LAB
  PMU102_Vm : rtlab/OpOutput  identifier_use=PMU102_Vm  identifier_hide=PMU102_Vm  nb_parents_identifier=0
      settings: SourceProductName=RT-LAB
  Spoofing attack : Subsystem
  Out1 : Outport  VectorParamsAs1DForOutWhenUnconnected=off
  wires:
  Demux/3 -> PMU102_I1m/1
  Demux/1 -> PMU102_Vm/1
  Demux/6 -> PMU102_I2a/1
  Demux/8 -> PMU102_I3a/1
  Demux/2 -> PMU102_Va/1
  Demux/7 -> PMU102_I3m/1
  Demux/4 -> PMU102_I1a/1
  Demux/5 -> PMU102_I2m/1
  In1/1 -> Spoofing attack/1(Input)
  Spoofing attack/1(Output) -> Out1/1, Demux/1

== system System_20220515/sm_master/PMU103_signals ==
  In1 : Inport
  Demux : Demux  Outputs=8
  PMU103_I1a : rtlab/OpOutput  identifier_use=PMU103_I1a  identifier_hide=PMU103_I1a  nb_parents_identifier=0
      settings: SourceProductName=RT-LAB
  PMU103_I1m : rtlab/OpOutput  identifier_use=PMU103_I1m  identifier_hide=PMU103_I1m  nb_parents_identifier=0
      settings: SourceProductName=RT-LAB
  PMU103_I2a : rtlab/OpOutput  identifier_use=PMU103_I2a  identifier_hide=PMU103_I2a  nb_parents_identifier=0
      settings: SourceProductName=RT-LAB
  PMU103_I2m : rtlab/OpOutput  identifier_use=PMU103_I2m  identifier_hide=PMU103_I2m  nb_parents_identifier=0
      settings: SourceProductName=RT-LAB
  PMU103_I3a : rtlab/OpOutput  identifier_use=PMU103_I3a  identifier_hide=PMU103_I3a  nb_parents_identifier=0
      settings: SourceProductName=RT-LAB
  PMU103_I3m : rtlab/OpOutput  identifier_use=PMU103_I3m  identifier_hide=PMU103_I3m  nb_parents_identifier=0
      settings: SourceProductName=RT-LAB
  PMU103_Va : rtlab/OpOutput  identifier_use=PMU103_Va  identifier_hide=PMU103_Va  nb_parents_identifier=0
      settings: SourceProductName=RT-LAB
  PMU103_Vm : rtlab/OpOutput  identifier_use=PMU103_Vm  identifier_hide=PMU103_Vm  nb_parents_identifier=0
      settings: SourceProductName=RT-LAB
  Spoofing attack : Subsystem
  Out1 : Outport  VectorParamsAs1DForOutWhenUnconnected=off
  wires:
  Demux/3 -> PMU103_I1m/1
  Demux/1 -> PMU103_Vm/1
  Demux/6 -> PMU103_I2a/1
  Demux/2 -> PMU103_Va/1
  Demux/4 -> PMU103_I1a/1
  Demux/5 -> PMU103_I2m/1
  In1/1 -> Spoofing attack/1(Input)
  Demux/7 -> PMU103_I3m/1
  Demux/8 -> PMU103_I3a/1
  Spoofing attack/1(Output) -> Out1/1, Demux/1

== system System_20220515/sm_master/PMU107_signals ==
  In1 : Inport
  Demux : Demux  Outputs=6
  PMU107_I1a : rtlab/OpOutput  identifier_use=PMU107_I1a  identifier_hide=PMU107_I1a  nb_parents_identifier=0
      settings: SourceProductName=RT-LAB
  PMU107_I1m : rtlab/OpOutput  identifier_use=PMU107_I1m  identifier_hide=PMU107_I1m  nb_parents_identifier=0
      settings: SourceProductName=RT-LAB
  PMU107_I2a : rtlab/OpOutput  identifier_use=PMU107_I2a  identifier_hide=PMU107_I2a  nb_parents_identifier=0
      settings: SourceProductName=RT-LAB
  PMU107_I2m : rtlab/OpOutput  identifier_use=PMU107_I2m  identifier_hide=PMU107_I2m  nb_parents_identifier=0
      settings: SourceProductName=RT-LAB
  PMU107_Va : rtlab/OpOutput  identifier_use=PMU107_Va  identifier_hide=PMU107_Va  nb_parents_identifier=0
      settings: SourceProductName=RT-LAB
  PMU107_Vm : rtlab/OpOutput  identifier_use=PMU107_Vm  identifier_hide=PMU107_Vm  nb_parents_identifier=0
      settings: SourceProductName=RT-LAB
  Spoofing attack : Subsystem
  Out1 : Outport  VectorParamsAs1DForOutWhenUnconnected=off
  wires:
  Demux/3 -> PMU107_I1m/1
  Demux/1 -> PMU107_Vm/1
  Demux/6 -> PMU107_I2a/1
  Demux/2 -> PMU107_Va/1
  Demux/4 -> PMU107_I1a/1
  Demux/5 -> PMU107_I2m/1
  In1/1 -> Spoofing attack/1(Input)
  Spoofing attack/1(Output) -> Out1/1, Demux/1

== system System_20220515/sm_master/PMU110_signals ==
  Input : Inport
  Demux : Demux  Outputs=12
  PMU110_I1a : rtlab/OpOutput  identifier_use=PMU110_I1a  identifier_hide=PMU110_I1a  nb_parents_identifier=0
      settings: SourceProductName=RT-LAB
  PMU110_I1m : rtlab/OpOutput  identifier_use=PMU110_I1m  identifier_hide=PMU110_I1m  nb_parents_identifier=0
      settings: SourceProductName=RT-LAB
  PMU110_I2a : rtlab/OpOutput  identifier_use=PMU110_I2a  identifier_hide=PMU110_I2a  nb_parents_identifier=0
      settings: SourceProductName=RT-LAB
  PMU110_I2m : rtlab/OpOutput  identifier_use=PMU110_I2m  identifier_hide=PMU110_I2m  nb_parents_identifier=0
      settings: SourceProductName=RT-LAB
  PMU110_I3a : rtlab/OpOutput  identifier_use=PMU110_I3a  identifier_hide=PMU110_I3a  nb_parents_identifier=0
      settings: SourceProductName=RT-LAB
  PMU110_I3m : rtlab/OpOutput  identifier_use=PMU110_I3m  identifier_hide=PMU110_I3m  nb_parents_identifier=0
      settings: SourceProductName=RT-LAB
  PMU110_I4a : rtlab/OpOutput  identifier_use=PMU110_I4a  identifier_hide=PMU110_I4a  nb_parents_identifier=0
      settings: SourceProductName=RT-LAB
  PMU110_I4m : rtlab/OpOutput  identifier_use=PMU110_I4m  identifier_hide=PMU110_I4m  nb_parents_identifier=0
      settings: SourceProductName=RT-LAB
  PMU110_I5a : rtlab/OpOutput  identifier_use=PMU110_I5a  identifier_hide=PMU110_I5a  nb_parents_identifier=0
      settings: SourceProductName=RT-LAB
  PMU110_I5m : rtlab/OpOutput  identifier_use=PMU110_I5m  identifier_hide=PMU110_I5m  nb_parents_identifier=0
      settings: SourceProductName=RT-LAB
  PMU110_Va : rtlab/OpOutput  identifier_use=PMU110_Va  identifier_hide=PMU110_Va  nb_parents_identifier=0
      settings: SourceProductName=RT-LAB
  PMU110_Vm : rtlab/OpOutput  identifier_use=PMU110_Vm  identifier_hide=PMU110_Vm  nb_parents_identifier=0
      settings: SourceProductName=RT-LAB
  Spoofing attack : Subsystem
  Output : Outport  VectorParamsAs1DForOutWhenUnconnected=off
  wires:
  Demux/1 -> PMU110_Vm/1
  Demux/2 -> PMU110_Va/1
  Demux/3 -> PMU110_I1m/1
  Demux/4 -> PMU110_I1a/1
  Demux/8 -> PMU110_I3a/1
  Demux/9 -> PMU110_I4m/1
  Demux/10 -> PMU110_I4a/1
  Demux/11 -> PMU110_I5m/1
  Demux/12 -> PMU110_I5a/1
  Demux/5 -> PMU110_I2m/1
  Demux/6 -> PMU110_I2a/1
  Demux/7 -> PMU110_I3m/1
  Input/1 -> Spoofing attack/1(Input)
  Spoofing attack/1(Output) -> Output/1, Demux/1

== system System_20220515/sm_master/PMU116_signals ==
  In1 : Inport
  Demux : Demux  Outputs=10
  PMU116_I1a : rtlab/OpOutput  identifier_use=PMU116_I1a  identifier_hide=PMU116_I1a  nb_parents_identifier=0
      settings: SourceProductName=RT-LAB
  PMU116_I1m : rtlab/OpOutput  identifier_use=PMU116_I1m  identifier_hide=PMU116_I1m  nb_parents_identifier=0
      settings: SourceProductName=RT-LAB
  PMU116_I2a : rtlab/OpOutput  identifier_use=PMU116_I2a  identifier_hide=PMU116_I2a  nb_parents_identifier=0
      settings: SourceProductName=RT-LAB
  PMU116_I2m : rtlab/OpOutput  identifier_use=PMU116_I2m  identifier_hide=PMU116_I2m  nb_parents_identifier=0
      settings: SourceProductName=RT-LAB
  PMU116_I3a : rtlab/OpOutput  identifier_use=PMU116_I3a  identifier_hide=PMU116_I3a  nb_parents_identifier=0
      settings: SourceProductName=RT-LAB
  PMU116_I3m : rtlab/OpOutput  identifier_use=PMU116_I3m  identifier_hide=PMU116_I3m  nb_parents_identifier=0
      settings: SourceProductName=RT-LAB
  PMU116_I4a : rtlab/OpOutput  identifier_use=PMU116_I4a  identifier_hide=PMU116_I4a  nb_parents_identifier=0
      settings: SourceProductName=RT-LAB
  PMU116_I4m : rtlab/OpOutput  identifier_use=PMU116_I4m  identifier_hide=PMU116_I4m  nb_parents_identifier=0
      settings: SourceProductName=RT-LAB
  PMU116_Va : rtlab/OpOutput  identifier_use=PMU116_Va  identifier_hide=PMU116_Va  nb_parents_identifier=0
      settings: SourceProductName=RT-LAB
  PMU116_Vm : rtlab/OpOutput  identifier_use=PMU116_Vm  identifier_hide=PMU116_Vm  nb_parents_identifier=0
      settings: SourceProductName=RT-LAB
  Spoofing attack : Subsystem
  Out1 : Outport  VectorParamsAs1DForOutWhenUnconnected=off
  wires:
  Demux/10 -> PMU116_I4a/1
  Demux/3 -> PMU116_I1m/1
  Demux/1 -> PMU116_Vm/1
  Demux/6 -> PMU116_I2a/1
  Demux/8 -> PMU116_I3a/1
  Demux/2 -> PMU116_Va/1
  Demux/7 -> PMU116_I3m/1
  Demux/4 -> PMU116_I1a/1
  Demux/5 -> PMU116_I2m/1
  Demux/9 -> PMU116_I4m/1
  In1/1 -> Spoofing attack/1(Input)
  Spoofing attack/1(Output) -> Demux/1, Out1/1

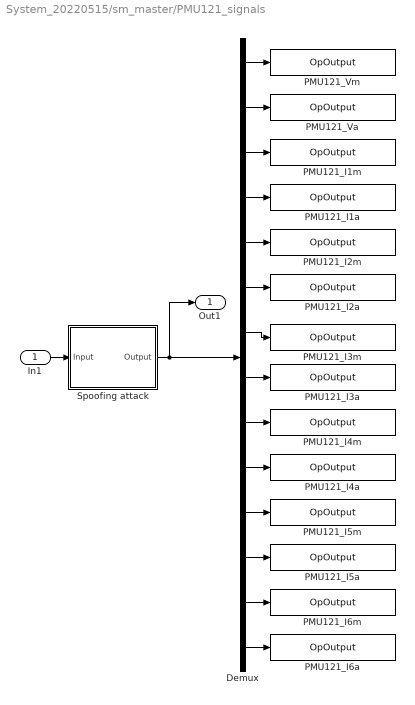
== system System_20220515/sm_master/PMU121_signals ==
  In1 : Inport
  Demux : Demux  Outputs=14
  PMU121_I1a : rtlab/OpOutput  identifier_use=PMU121_I1a  identifier_hide=PMU121_I1a  nb_parents_identifier=0
      settings: SourceProductName=RT-LAB
  PMU121_I1m : rtlab/OpOutput  identifier_use=PMU121_I1m  identifier_hide=PMU121_I1m  nb_parents_identifier=0
      settings: SourceProductName=RT-LAB
  PMU121_I2a : rtlab/OpOutput  identifier_use=PMU121_I2a  identifier_hide=PMU121_I2a  nb_parents_identifier=0
      settings: SourceProductName=RT-LAB
  PMU121_I2m : rtlab/OpOutput  identifier_use=PMU121_I2m  identifier_hide=PMU121_I2m  nb_parents_identifier=0
      settings: SourceProductName=RT-LAB
  PMU121_I3a : rtlab/OpOutput  identifier_use=PMU121_I3a  identifier_hide=PMU121_I3a  nb_parents_identifier=0
      settings: SourceProductName=RT-LAB
  PMU121_I3m : rtlab/OpOutput  identifier_use=PMU121_I3m  identifier_hide=PMU121_I3m  nb_parents_identifier=0
      settings: SourceProductName=RT-LAB
  PMU121_I4a : rtlab/OpOutput  identifier_use=PMU121_I4a  identifier_hide=PMU121_I4a  nb_parents_identifier=0
      settings: SourceProductName=RT-LAB
  PMU121_I4m : rtlab/OpOutput  identifier_use=PMU121_I4m  identifier_hide=PMU121_I4m  nb_parents_identifier=0
      settings: SourceProductName=RT-LAB
  PMU121_I5a : rtlab/OpOutput  identifier_use=PMU121_I5a  identifier_hide=PMU121_I5a  nb_parents_identifier=0
      settings: SourceProductName=RT-LAB
  PMU121_I5m : rtlab/OpOutput  identifier_use=PMU121_I5m  identifier_hide=PMU121_I5m  nb_parents_identifier=0
      settings: SourceProductName=RT-LAB
  PMU121_I6a : rtlab/OpOutput  identifier_use=PMU121_I6a  identifier_hide=PMU121_I6a  nb_parents_identifier=0
      settings: SourceProductName=RT-LAB
  PMU121_I6m : rtlab/OpOutput  identifier_use=PMU121_I6m  identifier_hide=PMU121_I6m  nb_parents_identifier=0
      settings: SourceProductName=RT-LAB
  PMU121_Va : rtlab/OpOutput  identifier_use=PMU121_Va  identifier_hide=PMU121_Va  nb_parents_identifier=0
      settings: SourceProductName=RT-LAB
  PMU121_Vm : rtlab/OpOutput  identifier_use=PMU121_Vm  identifier_hide=PMU121_Vm  nb_parents_identifier=0
      settings: SourceProductName=RT-LAB
  Spoofing attack : Subsystem
  Out1 : Outport  VectorParamsAs1DForOutWhenUnconnected=off
  wires:
  Demux/1 -> PMU121_Vm/1
  Demux/2 -> PMU121_Va/1
  In1/1 -> Spoofing attack/1(Input)
  Demux/3 -> PMU121_I1m/1
  Demux/4 -> PMU121_I1a/1
  Demux/8 -> PMU121_I3a/1
  Demux/9 -> PMU121_I4m/1
  Demux/10 -> PMU121_I4a/1
  Demux/11 -> PMU121_I5m/1
  Demux/12 -> PMU121_I5a/1
  Demux/13 -> PMU121_I6m/1
  Demux/14 -> PMU121_I6a/1
  Demux/5 -> PMU121_I2m/1
  Demux/6 -> PMU121_I2a/1
  Demux/7 -> PMU121_I3m/1
  Spoofing attack/1(Output) -> Out1/1, Demux/1

== system System_20220515/sm_master/PMU123_signals ==
  In1 : Inport
  Demux : Demux  Outputs=12
  PMU123_I1a : rtlab/OpOutput  identifier_use=PMU123_I1a  identifier_hide=PMU123_I1a  nb_parents_identifier=0
      settings: SourceProductName=RT-LAB
  PMU123_I1m : rtlab/OpOutput  identifier_use=PMU123_I1m  identifier_hide=PMU123_I1m  nb_parents_identifier=0
      settings: SourceProductName=RT-LAB
  PMU123_I2a : rtlab/OpOutput  identifier_use=PMU123_I2a  identifier_hide=PMU123_I2a  nb_parents_identifier=0
      settings: SourceProductName=RT-LAB
  PMU123_I2m : rtlab/OpOutput  identifier_use=PMU123_I2m  identifier_hide=PMU123_I2m  nb_parents_identifier=0
      settings: SourceProductName=RT-LAB
  PMU123_I3a : rtlab/OpOutput  identifier_use=PMU123_I3a  identifier_hide=PMU123_I3a  nb_parents_identifier=0
      settings: SourceProductName=RT-LAB
  PMU123_I3m : rtlab/OpOutput  identifier_use=PMU123_I3m  identifier_hide=PMU123_I3m  nb_parents_identifier=0
      settings: SourceProductName=RT-LAB
  PMU123_I4a : rtlab/OpOutput  identifier_use=PMU123_I4a  identifier_hide=PMU123_I4a  nb_parents_identifier=0
      settings: SourceProductName=RT-LAB
  PMU123_I4m : rtlab/OpOutput  identifier_use=PMU123_I4m  identifier_hide=PMU123_I4m  nb_parents_identifier=0
      settings: SourceProductName=RT-LAB
  PMU123_I5a : rtlab/OpOutput  identifier_use=PMU123_I5a  identifier_hide=PMU123_I5a  nb_parents_identifier=0
      settings: SourceProductName=RT-LAB
  PMU123_I5m : rtlab/OpOutput  identifier_use=PMU123_I5m  identifier_hide=PMU123_I5m  nb_parents_identifier=0
      settings: SourceProductName=RT-LAB
  PMU123_Va : rtlab/OpOutput  identifier_use=PMU123_Va  identifier_hide=PMU123_Va  nb_parents_identifier=0
      settings: SourceProductName=RT-LAB
  PMU123_Vm : rtlab/OpOutput  identifier_use=PMU123_Vm  identifier_hide=PMU123_Vm  nb_parents_identifier=0
      settings: SourceProductName=RT-LAB
  Spoofing attack : Subsystem
  Out1 : Outport  VectorParamsAs1DForOutWhenUnconnected=off
  wires:
  Demux/1 -> PMU123_Vm/1
  Demux/2 -> PMU123_Va/1
  Demux/3 -> PMU123_I1m/1
  Demux/4 -> PMU123_I1a/1
  Demux/8 -> PMU123_I3a/1
  Demux/9 -> PMU123_I4m/1
  Demux/10 -> PMU123_I4a/1
  Demux/11 -> PMU123_I5m/1
  Demux/12 -> PMU123_I5a/1
  Demux/5 -> PMU123_I2m/1
  Demux/6 -> PMU123_I2a/1
  Demux/7 -> PMU123_I3m/1
  In1/1 -> Spoofing attack/1(Input)
  Spoofing attack/1(Output) -> Out1/1, Demux/1
